simulink model "ds_capital_nonlinear_1o_wo_simulation_simu"  (R2022b)
settings: Solver=FixedStepAuto  StartTime=0.0  StopTime=N*time_step  FixedStep=5  RelTol=1e-3
values from neighbouring files (symbols this model uses):
  A = temp.A    [ds_capital_nonlinear_1o_wo_simulation.m]    (also in ds_capital_nonlinear_1o_wo_simulation_data.mat = 1)
  B = temp.B    [ds_capital_nonlinear_1o_wo_simulation.m]    (also in ds_capital_nonlinear_1o_wo_simulation_data.mat = [0.0152043019802 0.0152043019802 0.0152043019802 0.015204301)
  C = temp.C    [ds_capital_nonlinear_1o_wo_simulation.m]    (also in ds_capital_nonlinear_1o_wo_simulation_data.mat = 0.125)
  D = temp.D    [ds_capital_nonlinear_1o_wo_simulation.m]    (also in ds_capital_nonlinear_1o_wo_simulation_data.mat = [0 0 0 0 0 0])
  OR = [0.65 1 9.81 0.5 0]    [ds_capital_nonlinear_1o_wo_simulation_data.mat]
settings Model: Creator=chuan  LastModifiedBy=chuan

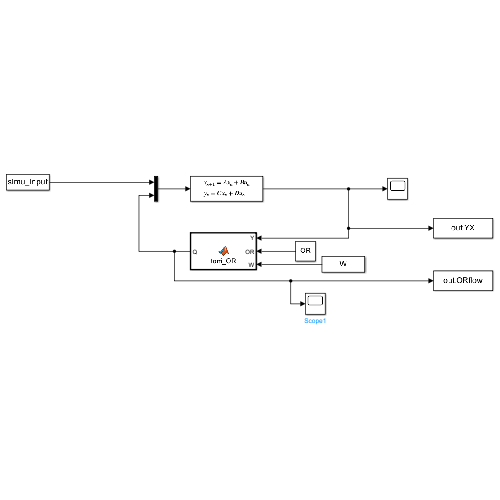
[thumbnail: Simulink's stored preview of the top-level diagram]
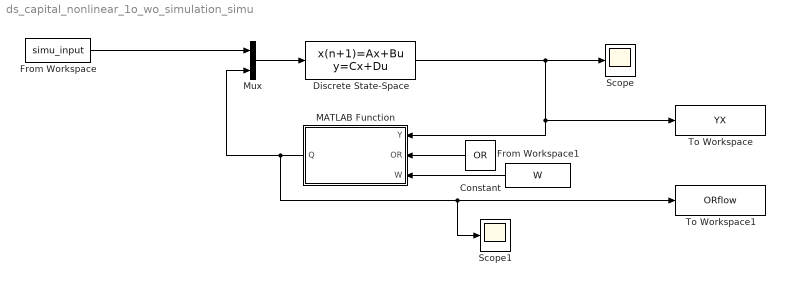
== system ds_capital_nonlinear_1o_wo_simulation_simu ==
  Constant : Constant  Value=OR
  Discrete State-Space : DiscreteStateSpace  A=A  B=B  C=C  D=D  SampleTime=-1
  From Workspace : FromWorkspace  VariableName=simu_input  SampleTime=-1
  From Workspace1 : FromWorkspace  VariableName=W  SampleTime=-1
  MATLAB Function : MATLAB Function  TreatAsAtomicUnit=on
  Mux : Mux  Inputs=2
  Scope : Scope
  Scope1 : Scope
  To Workspace : ToWorkspace  VariableName=YX  SaveFormat=Timeseries  SampleTime=-1
  To Workspace1 : ToWorkspace  VariableName=ORflow  SaveFormat=Timeseries  SampleTime=-1
  wires:
  Discrete State-Space/1 -> MATLAB Function/1(Y), To Workspace/1, Scope/1
  Mux/1 -> Discrete State-Space/1
  Constant/1 -> MATLAB Function/2(OR)
  MATLAB Function/1(Q) -> Mux/2, Scope1/1, To Workspace1/1
  From Workspace/1 -> Mux/1
  From Workspace1/1 -> MATLAB Function/3(W)

== matlab function ds_capital_nonlinear_1o_wo_simulation_simu/MATLAB Function ==
  data: Y input; Q output; OR input; W input
function Q = torri_OR(Y,OR,W)

% Import Orifice Data
Cd = OR(1);
A0 = OR(2);
g = OR(3);
Yfull = OR(4);
Z0 = OR(5);

% Compute real area opening
A0 = W*A0;

% Compute Outflow
constant = sqrt(32/27);
boundary = 0.25*(3*W*Yfull + 4*Z0);

% constant = 1;
% boundary = Yfull + Z0;

% Compute Outflow
if Y <= Z0
        Q = 0;
    elseif Y > Z0 && Y < boundary
        if W ~= 0 
            CwL = (Cd*A0*sqrt(g))/(W*Yfull);
            CwL = constant*CwL;
            Q = CwL*(Y-Z0)^(1.5);
        else
            Q = 0;
        end
    else
        He = Y-(Z0 + W*Yfull/2);
        Q = Cd*A0*sqrt(2*g*He);
end

if W == 0
    Q = 0;
end

end
